simulink model "secon_example2"  (Simulink 8.7)
settings: Solver=ode45  StartTime=0.0  StopTime=100  RelTol=1e-3
libraries: simulink x1, fuzblock x1
settings Model: Creator=home2  LastModifiedBy=mohamed
settings DataIOCC: SignalLoggingSaveFormat=ModelDataLogs
settings DebuggingCC: SolverPrmCheckMsg=warning  FcnCallInpInsideContextMsg=UseLocalSettings  StateNameClashWarn=warning
settings GRTTargetCC: CombineOutputUpdateFcns=off  GRTInterface=on

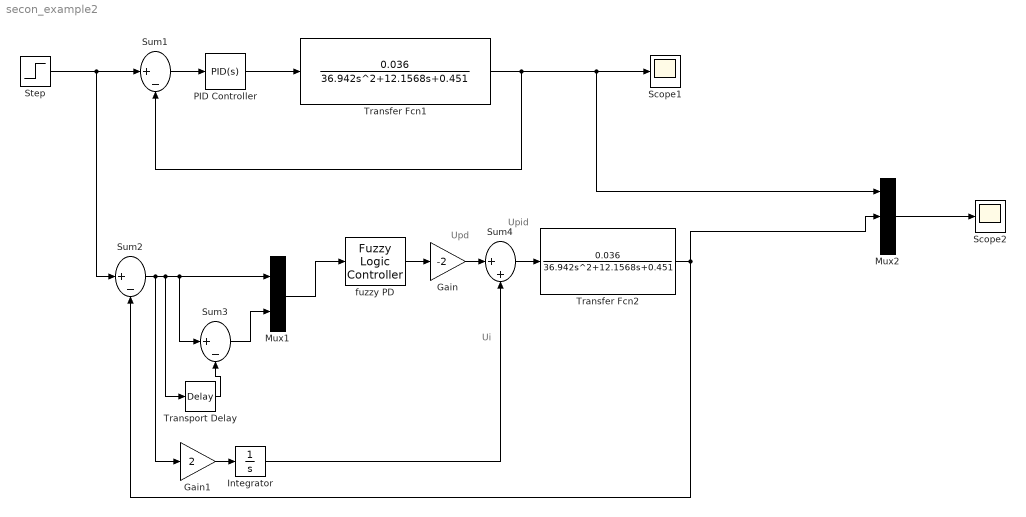
== system secon_example2 ==
  note: Upd
  note: Ui
  note: Upid
  Gain : Gain  Gain=-2
  Gain1 : Gain  Gain=2
  Integrator : Integrator
  Mux1 : Mux  Inputs=2
  Mux2 : Mux  Inputs=3
  PID Controller : simulink/Continuous/PID Controller  Controller=PID  TimeDomain=Continuous-time  SampleTime=-1  IntegratorMethod=Forward Euler  FilterMethod=Forward Euler  Form=Parallel  UseFilter=on  ControllerParametersSource=internal  P=90  I=4  D=7  N=30  InitialConditionSource=internal  InitialConditionForIntegrator=0  InitialConditionForFilter=0  ExternalReset=none  LimitOutput=off  UpperSaturationLimit=inf  LowerSaturationLimit=-inf  LinearizeAsGain=on  AntiWindupMode=none  Kb=1  TrackingMode=off  Kt=1  PParamMin=[]  PParamMax=[]  IParamMin=[]  IParamMax=[]  DParamMin=[]  DParamMax=[]  NParamMin=[]  NParamMax=[]  KbParamMin=[]  KbParamMax=[]  KtParamMin=[]  KtParamMax=[]  POutMin=[]  POutMax=[]  IOutMin=[]  IOutMax=[]  DOutMin=[]  DOutMax=[]  NOutMin=[]  NOutMax=[]  KbOutMin=[]  KbOutMax=[]  KtOutMin=[]  KtOutMax=[]  IntegratorOutMin=[]  IntegratorOutMax=[]  FilterOutMin=[]  FilterOutMax=[]  SumOutMin=[]  SumOutMax=[]  SumI1OutMin=[]  SumI1OutMax=[]  SumI2OutMin=[]  SumI2OutMax=[]  SumI3OutMin=[]  SumI3OutMax=[]  SumDOutMin=[]  SumDOutMax=[]  SaturationOutMin=[]  SaturationOutMax=[]  IntegratorContinuousStateAttributes=''  IntegratorStateMustResolveToSignalObject=off  IntegratorRTWStateStorageClass=Auto  FilterContinuousStateAttributes=''  FilterStateMustResolveToSignalObject=off  FilterRTWStateStorageClass=Auto  DifferentiatorICPrevScaledInput=0  DifferentiatorOutMin=[]  DifferentiatorOutMax=[]
  Scope1 : Scope
  Scope2 : Scope
  Step : Step  Time=0  SampleTime=0
  Sum1 : Sum  Inputs=|+-
  Sum2 : Sum  Inputs=|+-
  Sum3 : Sum  Inputs=|+-
  Sum4 : Sum  Inputs=|++
  Transfer Fcn1 : TransferFcn  Numerator=[0.036]  Denominator=[36.942 12.1568 0.451]
  Transfer Fcn2 : TransferFcn  Numerator=[0.036]  Denominator=[36.942 12.1568 0.451]
  Transport Delay : TransportDelay
  fuzzy PD : fuzblock/Fuzzy Logic  Controller  fis=ex2
  wires:
  PID Controller/1 -> Transfer Fcn1/1
  Sum1/1 -> PID Controller/1
  Transfer Fcn2/1 -> Sum2/2, Mux2/2
  Step/1 -> Sum2/1, Sum1/1
  Transport Delay/1 -> Sum3/2
  Sum3/1 -> Mux1/2
  Mux1/1 -> fuzzy PD/1
  Sum2/1 -> Transport Delay/1, Mux1/1, Sum3/1, Gain1/1
  fuzzy PD/1 -> Gain/1
  Gain1/1 -> Integrator/1
  Sum4/1 -> Transfer Fcn2/1
  Gain/1 -> Sum4/1
  Integrator/1 -> Sum4/2
  Transfer Fcn1/1 -> Sum1/2, Mux2/1, Scope1/1
  Mux2/1 -> Scope2/1
